simulink model "m02_PMSM_HDL"  (R2023b)
settings: Solver=FixedStepDiscrete  StartTime=0.0  StopTime=0.6  RelTol=1e-3  AbsTol=1e-3
PreLoadFcn:
  | control_data;
  | pmsm_data;
  | 
  | avgFactor = 1;
undefined symbols (not defined in the file): ee_sli_rtmsupport, f1478573793584, f1859323186544, fsw, gcbh, J, Ld, Lq, N, PM, Pmax, Tmax, Ts, Tsc
libraries: hdlssclib x24, simulink x8, SimscapeFPGAHIL_lib x6, fpga_utils_lib x5, hdlsllib x4, eeTransforms x2, eePwmGeneratorTwoLevel x1, eePmsmCurrentController x1, eePmsmCurrentReferenceGen x1, eeVelocityController x1
(part 2 of 3)

== system m02_PMSM_HDL/FPGA Model/HDL Plant/Pejovic HDL Plant/HDL Subsystem/HDL Algorithm/Output ==
  U : Inport
  State : Inport  Port=2
  t : Inport  Port=3
  Mode : Inport  Port=4
  network_outputs : Subsystem
  State Out : Outport  VectorParamsAs1DForOutWhenUnconnected=off
  wires:
  State/1 -> network_outputs/1(x)
  U/1 -> network_outputs/2(u)
  network_outputs/1(vs) -> State Out/1
  t/1 -> network_outputs/3(t)
  Mode/1 -> network_outputs/4(m)

== system m02_PMSM_HDL/FPGA Model/HDL Plant/Pejovic HDL Plant/HDL Subsystem/HDL Algorithm/State Update ==
  U : Inport
  t : Inport  Port=2
  Algebraic Clump1 : Subsystem
  Algebraic Clump2 : Subsystem
  Algebraic Clump3 : Subsystem
  Algebraic Clump4 : Subsystem
  Differential Clump : Subsystem
  Initial Conditions : Subsystem
  State : Outport  VectorParamsAs1DForOutWhenUnconnected=off
  Mode : Outport  Port=2  VectorParamsAs1DForOutWhenUnconnected=off
  wires:
  Initial Conditions/1(State Out) -> Differential Clump/2(State), State/1
  Initial Conditions/2(Mode Out) -> Mode/1, Differential Clump/3(Mode Vector)
  t/1 -> Algebraic Clump1/4(t), Algebraic Clump2/4(t), Algebraic Clump4/4(t), Algebraic Clump3/4(t), Differential Clump/4(t)
  U/1 -> Algebraic Clump1/1(U), Algebraic Clump2/1(U), Algebraic Clump3/1(U), Algebraic Clump4/1(U), Differential Clump/1(U)
  Differential Clump/1(State Out) -> Algebraic Clump1/2(State)
  Differential Clump/2(Mode Vector Out) -> Algebraic Clump1/3(Mode Vector)
  Algebraic Clump1/1(State Out) -> Algebraic Clump2/2(State)
  Algebraic Clump1/2(Mode Vector Out) -> Algebraic Clump2/3(Mode Vector)
  Algebraic Clump2/2(Mode Vector Out) -> Algebraic Clump3/3(Mode Vector)
  Algebraic Clump2/1(State Out) -> Algebraic Clump3/2(State)
  Algebraic Clump3/1(State Out) -> Algebraic Clump4/2(State)
  Algebraic Clump3/2(Mode Vector Out) -> Algebraic Clump4/3(Mode Vector)
  Algebraic Clump4/2(Mode Vector Out) -> Initial Conditions/2(Mode)
  Algebraic Clump4/1(State Out) -> Initial Conditions/1(State)

== system m02_PMSM_HDL/FPGA Model/HDL Plant/Standard HDL Plant/HDL Subsystem/HDL Algorithm/Clock ==
  Delay : Delay  DelayLength=1
  Sample Time : Constant  Value=single(2.5e-06)  OutDataTypeStr=single  SampleTime=2.5e-06
  Sum : Sum  OutDataTypeStr=single
  t : Outport  VectorParamsAs1DForOutWhenUnconnected=off
  wires:
  Sample Time/1 -> Sum/1
  Sum/1 -> Delay/1
  Delay/1 -> t/1, Sum/2

== system m02_PMSM_HDL/FPGA Model/HDL Plant/Standard HDL Plant/HDL Subsystem/HDL Algorithm/Output ==
  U : Inport
  State : Inport  Port=2
  t : Inport  Port=3
  Mode : Inport  Port=4
  network_outputs : Subsystem
  State Out : Outport  VectorParamsAs1DForOutWhenUnconnected=off
  wires:
  Mode/1 -> network_outputs/4(m)
  t/1 -> network_outputs/3(t)
  State/1 -> network_outputs/1(x)
  U/1 -> network_outputs/2(u)
  network_outputs/1(vs) -> State Out/1

== system m02_PMSM_HDL/FPGA Model/HDL Plant/Standard HDL Plant/HDL Subsystem/HDL Algorithm/State Update ==
  U : Inport
  t : Inport  Port=2
  Algebraic Clump1 : Subsystem
  Algebraic Clump2 : Subsystem
  Algebraic Clump3 : Subsystem
  Algebraic Clump4 : Subsystem
  Data Type Conversion : DataTypeConversion  OutDataTypeStr=int32  RndMeth=Nearest  SaturateOnIntegerOverflow=off
  Differential Clump : Subsystem
  Initial Conditions : Subsystem
  Mode Assignment : Assignment  IndexOptions=Index vector (dialog)  Indices="[1  2  4  5  3  6]"  OutputSizes=1
  network_modes : Subsystem
  State : Outport  VectorParamsAs1DForOutWhenUnconnected=off
  Mode : Outport  Port=2  VectorParamsAs1DForOutWhenUnconnected=off
  wires:
  U/1 -> Algebraic Clump3/1(U), Algebraic Clump4/1(U), Algebraic Clump2/1(U), Algebraic Clump1/1(U), network_modes/2(u), Differential Clump/1(U)
  t/1 -> Algebraic Clump3/4(t), Algebraic Clump4/4(t), Algebraic Clump2/4(t), Algebraic Clump1/4(t), network_modes/3(t), Differential Clump/4(t)
  network_modes/1(vs) -> Data Type Conversion/1
  Initial Conditions/1(State Out) -> State/1, Differential Clump/2(State)
  Data Type Conversion/1 -> Mode Assignment/2
  Initial Conditions/2(Mode Out) -> Mode/1, Differential Clump/3(Mode Vector)
  Mode Assignment/1 -> Algebraic Clump1/3(Mode Vector)
  Differential Clump/1(State Out) -> network_modes/1(x), Algebraic Clump1/2(State)
  Differential Clump/2(Mode Vector Out) -> Mode Assignment/1
  Algebraic Clump4/2(Mode Vector Out) -> Initial Conditions/2(Mode)
  Algebraic Clump4/1(State Out) -> Initial Conditions/1(State)
  Algebraic Clump1/1(State Out) -> Algebraic Clump2/2(State)
  Algebraic Clump1/2(Mode Vector Out) -> Algebraic Clump2/3(Mode Vector)
  Algebraic Clump2/2(Mode Vector Out) -> Algebraic Clump3/3(Mode Vector)
  Algebraic Clump2/1(State Out) -> Algebraic Clump3/2(State)
  Algebraic Clump3/1(State Out) -> Algebraic Clump4/2(State)
  Algebraic Clump3/2(Mode Vector Out) -> Algebraic Clump4/3(Mode Vector)

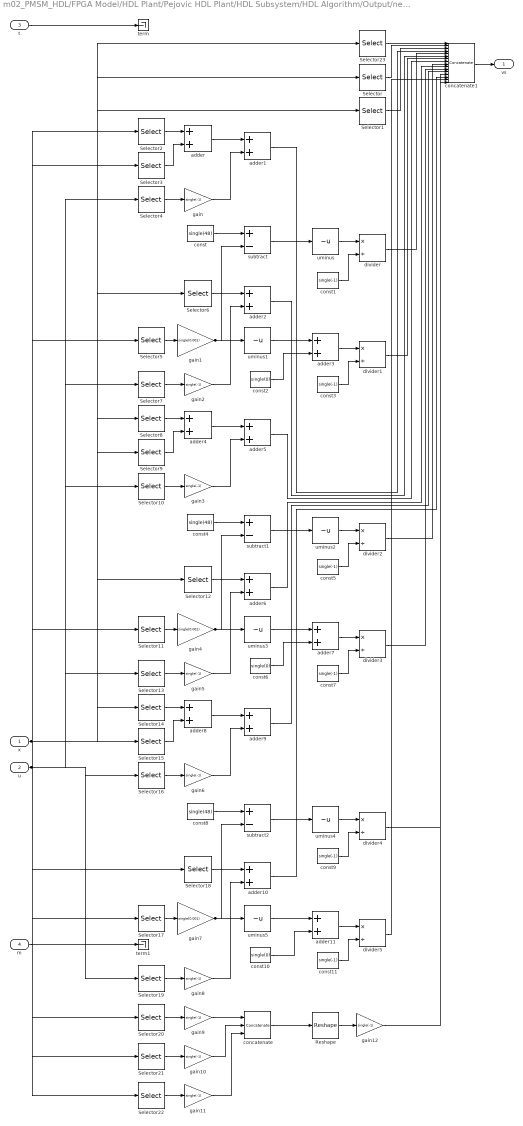
== system m02_PMSM_HDL/FPGA Model/HDL Plant/Pejovic HDL Plant/HDL Subsystem/HDL Algorithm/Output/network_outputs ==
  x : Inport  OutDataTypeStr=single  PortDimensions=[12 1]  SampleTime=2.5e-06
  u : Inport  Port=2  OutDataTypeStr=single  PortDimensions=[6 1]  SampleTime=2.5e-06
  t : Inport  Port=3  OutDataTypeStr=single  SampleTime=2.5e-06
  m : Inport  Port=4  OutDataTypeStr=int32  SampleTime=2.5e-06
  Reshape : Reshape  OutputDimensionality=Row vector (2-D)
  Selector : Selector  SampleTime=2.5e-06  IndexOptions=Index vector (dialog)  Indices=double(7)  OutputSizes=double(0)
  Selector1 : Selector  SampleTime=2.5e-06  IndexOptions=Index vector (dialog)  Indices=double(9)  OutputSizes=double(0)
  Selector{8,10..13} (5 alike) : Selector  SampleTime=2.5e-06  IndexOptions=Index vector (dialog)  Indices=double(2)  OutputSizes=double(0)
  Selector{14,16..19} (5 alike) : Selector  SampleTime=2.5e-06  IndexOptions=Index vector (dialog)  Indices=double(3)  OutputSizes=double(0)
  Selector15 : Selector  SampleTime=2.5e-06  IndexOptions=Index vector (dialog)  Indices=double(6)  OutputSizes=double(0)
  Selector{2,4..7} (5 alike) : Selector  SampleTime=2.5e-06  IndexOptions=Index vector (dialog)  Indices=double(1)  OutputSizes=double(0)
  Selector20 : Selector  SampleTime=2.5e-06  IndexOptions=Index vector (dialog)  Indices=double(4)  OutputSizes=double(0)
  Selector21 : Selector  SampleTime=2.5e-06  IndexOptions=Index vector (dialog)  Indices=double(5)  OutputSizes=double(0)
  Selector22 : Selector  SampleTime=2.5e-06  IndexOptions=Index vector (dialog)  Indices=double(6)  OutputSizes=double(0)
  Selector23 : Selector  SampleTime=2.5e-06  IndexOptions=Index vector (dialog)  Indices=double(8)  OutputSizes=double(0)
  Selector3 : Selector  SampleTime=2.5e-06  IndexOptions=Index vector (dialog)  Indices=double(4)  OutputSizes=double(0)
  Selector9 : Selector  SampleTime=2.5e-06  IndexOptions=Index vector (dialog)  Indices=double(5)  OutputSizes=double(0)
  adder{,1..11} (12 alike) : Sum  OutDataTypeStr=single  AccumDataTypeStr=single  SampleTime=2.5e-06
  concatenate : Concatenate  NumInputs=3  Mode=Multidimensional array
  concatenate1 : Concatenate  NumInputs=16  Mode=Multidimensional array  ConcatenateDimension=2
  const : Constant  Value=single(48)  VectorParams1D=off  OutDataTypeStr=single  SampleTime=2.5e-06
  const{1,3,5,7,9,11} (6 alike) : Constant  Value=single(-1)  VectorParams1D=off  OutDataTypeStr=single  SampleTime=2.5e-06
  const10 : Constant  Value=single(0)  VectorParams1D=off  OutDataTypeStr=single  SampleTime=2.5e-06
  const2 : Constant  Value=single(0)  VectorParams1D=off  OutDataTypeStr=single  SampleTime=2.5e-06
  const4 : Constant  Value=single(48)  VectorParams1D=off  OutDataTypeStr=single  SampleTime=2.5e-06
  const6 : Constant  Value=single(0)  VectorParams1D=off  OutDataTypeStr=single  SampleTime=2.5e-06
  const8 : Constant  Value=single(48)  VectorParams1D=off  OutDataTypeStr=single  SampleTime=2.5e-06
  divider{,1..5} (6 alike) : Product  Inputs=*/  OutDataTypeStr=single  SampleTime=2.5e-06
  gain{,2..3,5..6,8..12} (10 alike) : Gain  Gain=single(-1)  OutDataTypeStr=single  SampleTime=2.5e-06
  gain1 : Gain  Gain=single(0.001)  OutDataTypeStr=single  SampleTime=2.5e-06
  gain4 : Gain  Gain=single(0.001)  OutDataTypeStr=single  SampleTime=2.5e-06
  gain7 : Gain  Gain=single(0.001)  OutDataTypeStr=single  SampleTime=2.5e-06
  subtract : Sum  Inputs=+-  OutDataTypeStr=single  AccumDataTypeStr=single  SampleTime=2.5e-06
  subtract1 : Sum  Inputs=+-  OutDataTypeStr=single  AccumDataTypeStr=single  SampleTime=2.5e-06
  subtract2 : Sum  Inputs=+-  OutDataTypeStr=single  AccumDataTypeStr=single  SampleTime=2.5e-06
  term : Terminator
  term1 : Terminator
  uminus{,1..5} (6 alike) : UnaryMinus  SampleTime=2.5e-06
  vs : Outport  OutDataTypeStr=single  PortDimensions=[1 18]  SampleTime=2.5e-06
  wires:
  Selector20/1 -> gain9/1
  Selector2/1 -> adder/1
  t/1 -> term/1
  u/1 -> Selector19/1, Selector16/1, Selector10/1, Selector7/1, Selector13/1, Selector4/1
  x/1 -> Selector6/1, Selector12/1, Selector1/1, Selector/1, Selector18/1, Selector22/1, Selector21/1, Selector20/1, Selector23/1, Selector15/1, Selector5/1, Selector9/1, Selector14/1, Selector2/1, Selector3/1, Selector11/1, Selector17/1, Selector8/1
  m/1 -> term1/1
  Selector3/1 -> adder/2
  Selector4/1 -> gain/1
  Selector5/1 -> gain1/1
  Selector6/1 -> adder2/1
  Selector7/1 -> gain2/1
  Selector9/1 -> adder4/2
  Selector8/1 -> adder4/1
  Selector11/1 -> gain4/1
  Selector10/1 -> gain3/1
  Selector12/1 -> adder6/1
  Selector13/1 -> gain5/1
  Selector15/1 -> adder8/2
  Selector14/1 -> adder8/1
  Selector17/1 -> gain7/1
  Selector16/1 -> gain6/1
  Selector18/1 -> adder10/1
  Selector19/1 -> gain8/1
  Selector22/1 -> gain11/1
  Selector21/1 -> gain10/1
  adder/1 -> adder1/1
  gain1/1 -> uminus1/1, subtract/2
  gain/1 -> adder1/2
  const1/1 -> divider/2
  const10/1 -> adder11/2
  const/1 -> subtract/1
  gain2/1 -> adder2/2
  adder5/1 -> concatenate1/8
  adder4/1 -> adder5/1
  gain4/1 -> uminus3/1, subtract1/2
  gain3/1 -> adder5/2
  const3/1 -> divider1/2
  const2/1 -> adder3/2
  const4/1 -> subtract1/1
  gain6/1 -> adder9/2
  gain5/1 -> adder6/2
  adder9/1 -> concatenate1/12
  adder8/1 -> adder9/1
  const6/1 -> adder7/2
  const8/1 -> subtract2/1
  gain8/1 -> adder10/2
  gain7/1 -> uminus5/1, subtract2/2
  subtract/1 -> uminus/1
  gain9/1 -> concatenate/1
  gain11/1 -> concatenate/3
  gain10/1 -> concatenate/2
  adder1/1 -> concatenate1/4
  adder2/1 -> concatenate1/6
  uminus2/1 -> divider2/1
  uminus1/1 -> adder3/1
  subtract1/1 -> uminus2/1
  adder6/1 -> concatenate1/10
  uminus3/1 -> adder7/1
  uminus/1 -> divider/1
  subtract2/1 -> uminus4/1
  adder10/1 -> concatenate1/14
  uminus5/1 -> adder11/1
  concatenate/1 -> Reshape/1
  adder3/1 -> divider1/1
  const5/1 -> divider2/2
  adder7/1 -> divider3/1
  const7/1 -> divider3/2
  uminus4/1 -> divider4/1
  const9/1 -> divider4/2
  adder11/1 -> divider5/1
  const11/1 -> divider5/2
  Reshape/1 -> gain12/1
  Selector23/1 -> concatenate1/1
  Selector/1 -> concatenate1/2
  Selector1/1 -> concatenate1/3
  divider/1 -> concatenate1/5
  divider1/1 -> concatenate1/7
  divider2/1 -> concatenate1/9
  divider3/1 -> concatenate1/11
  divider4/1 -> concatenate1/13
  divider5/1 -> concatenate1/15
  gain12/1 -> concatenate1/16
  concatenate1/1 -> vs/1

== system m02_PMSM_HDL/FPGA Model/HDL Plant/Pejovic HDL Plant/HDL Subsystem/HDL Algorithm/State Update/Algebraic Clump1 ==
  U : Inport
  State : Inport  Port=2
  Mode Vector : Inport  Port=3
  t : Inport  Port=4
  Default Index : Constant  Value=fi(0,0,2,0)  SampleTime=2.5e-06
  Multiply F : hdlssclib/NFPSparseConstMultiply  constMatrix=single(f1478573793584.ClumpInfo(1).MdInv)  MatrixType=single  PropDataType=single  defWL=48
  Multiply State : hdlssclib/NFPSparseConstMultiply  constMatrix=single(f1478573793584.ClumpInfo(1).Ad)  MatrixType=single  PropDataType=single  defWL=48
  Out States : Selector  IndexOptions=Index vector (dialog)  Indices="[1  2  3  4]"  OutputSizes=1
  Output Sum : Sum  Inputs=+-
  Owned States : Selector  IndexOptions=Index vector (dialog)  Indices="[1  2  3  4]"  OutputSizes=1
  Ref Inputs : Selector  IndexOptions=Index vector (dialog)  Indices=[1]  OutputSizes=1
  Ref Modes : Selector  IndexOptions=Index vector (dialog)  Indices=[1]  OutputSizes=1
  Ref States : Selector  IndexOptions=Index vector (dialog)  Indices="[7   8   9  10  11  12]"  OutputSizes=1
  State Assign : Assignment  IndexOptions=Index vector (dialog)  Indices="[7   8   9  10]"  OutputSizes=1
  extClump0_F : Subsystem
  transpose : Math  Operator=transpose  SignedPower=on  RndMeth=Zero
  State Out : Outport  VectorParamsAs1DForOutWhenUnconnected=off
  Mode Vector Out : Outport  Port=2  VectorParamsAs1DForOutWhenUnconnected=off
  wires:
  State/1 -> Ref States/1, State Assign/1
  Mode Vector/1 -> Mode Vector Out/1, Ref Modes/1
  U/1 -> Ref Inputs/1
  Ref States/1 -> extClump0_F/1(x), Owned States/1
  Ref Inputs/1 -> extClump0_F/2(u)
  Ref Modes/1 -> extClump0_F/4(m)
  t/1 -> extClump0_F/3(t)
  Owned States/1 -> Multiply State/1
  State Assign/1 -> State Out/1
  Out States/1 -> State Assign/2
  extClump0_F/1(vs) -> transpose/1
  transpose/1 -> Multiply F/1
  Default Index/1 -> Multiply State/2, Multiply F/2
  Multiply State/1 -> Output Sum/1
  Multiply F/1 -> Output Sum/2
  Output Sum/1 -> Out States/1

== system m02_PMSM_HDL/FPGA Model/HDL Plant/Pejovic HDL Plant/HDL Subsystem/HDL Algorithm/State Update/Algebraic Clump2 ==
  U : Inport
  State : Inport  Port=2
  Mode Vector : Inport  Port=3
  t : Inport  Port=4
  Default Index : Constant  Value=fi(0,0,2,0)  SampleTime=2.5e-06
  Multiply F : hdlssclib/NFPSparseConstMultiply  constMatrix=single(f1478573793584.ClumpInfo(2).MdInv)  MatrixType=single  PropDataType=single  defWL=48
  Multiply State : hdlssclib/NFPSparseConstMultiply  constMatrix=single(f1478573793584.ClumpInfo(2).Ad)  MatrixType=single  PropDataType=single  defWL=48
  Out States : Selector  IndexOptions=Index vector (dialog)  Indices="[1  2]"  OutputSizes=1
  Output Sum : Sum  Inputs=+-
  Owned States : Selector  IndexOptions=Index vector (dialog)  Indices="[1  2]"  OutputSizes=1
  Ref Inputs : Selector  IndexOptions=Index vector (dialog)  Indices="[6  3]"  OutputSizes=1
  Ref Modes : Selector  IndexOptions=Index vector (dialog)  Indices=[1]  OutputSizes=1
  Ref States : Selector  IndexOptions=Index vector (dialog)  Indices="[3   6  10  11  12]"  OutputSizes=1
  State Assign : Assignment  IndexOptions=Index vector (dialog)  Indices="[3  6]"  OutputSizes=1
  extClump1_F : Subsystem
  transpose : Math  Operator=transpose  SignedPower=on  RndMeth=Zero
  State Out : Outport  VectorParamsAs1DForOutWhenUnconnected=off
  Mode Vector Out : Outport  Port=2  VectorParamsAs1DForOutWhenUnconnected=off
  wires:
  State/1 -> Ref States/1, State Assign/1
  Out States/1 -> State Assign/2
  U/1 -> Ref Inputs/1
  Mode Vector/1 -> Mode Vector Out/1, Ref Modes/1
  Ref States/1 -> extClump1_F/1(x), Owned States/1
  Ref Inputs/1 -> extClump1_F/2(u)
  Ref Modes/1 -> extClump1_F/4(m)
  t/1 -> extClump1_F/3(t)
  Owned States/1 -> Multiply State/1
  extClump1_F/1(vs) -> transpose/1
  transpose/1 -> Multiply F/1
  Default Index/1 -> Multiply State/2, Multiply F/2
  Multiply State/1 -> Output Sum/1
  Multiply F/1 -> Output Sum/2
  Output Sum/1 -> Out States/1
  State Assign/1 -> State Out/1

== system m02_PMSM_HDL/FPGA Model/HDL Plant/Pejovic HDL Plant/HDL Subsystem/HDL Algorithm/State Update/Algebraic Clump3 ==
  U : Inport
  State : Inport  Port=2
  Mode Vector : Inport  Port=3
  t : Inport  Port=4
  Default Index : Constant  Value=fi(0,0,2,0)  SampleTime=2.5e-06
  Multiply F : hdlssclib/NFPSparseConstMultiply  constMatrix=single(f1478573793584.ClumpInfo(3).MdInv)  MatrixType=single  PropDataType=single  defWL=48
  Multiply State : hdlssclib/NFPSparseConstMultiply  constMatrix=single(f1478573793584.ClumpInfo(3).Ad)  MatrixType=single  PropDataType=single  defWL=48
  Out States : Selector  IndexOptions=Index vector (dialog)  Indices="[1  2]"  OutputSizes=1
  Output Sum : Sum  Inputs=+-
  Owned States : Selector  IndexOptions=Index vector (dialog)  Indices="[1  2]"  OutputSizes=1
  Ref Inputs : Selector  IndexOptions=Index vector (dialog)  Indices="[5  2]"  OutputSizes=1
  Ref Modes : Selector  IndexOptions=Index vector (dialog)  Indices=[1]  OutputSizes=1
  Ref States : Selector  IndexOptions=Index vector (dialog)  Indices="[2   5  10  11  12]"  OutputSizes=1
  State Assign : Assignment  IndexOptions=Index vector (dialog)  Indices="[2  5]"  OutputSizes=1
  extClump2_F : Subsystem
  transpose : Math  Operator=transpose  SignedPower=on  RndMeth=Zero
  State Out : Outport  VectorParamsAs1DForOutWhenUnconnected=off
  Mode Vector Out : Outport  Port=2  VectorParamsAs1DForOutWhenUnconnected=off
  wires:
  Output Sum/1 -> Out States/1
  Default Index/1 -> Multiply State/2, Multiply F/2
  State/1 -> State Assign/1, Ref States/1
  State Assign/1 -> State Out/1
  U/1 -> Ref Inputs/1
  Ref Inputs/1 -> extClump2_F/2(u)
  Mode Vector/1 -> Ref Modes/1, Mode Vector Out/1
  Ref States/1 -> extClump2_F/1(x), Owned States/1
  Owned States/1 -> Multiply State/1
  Ref Modes/1 -> extClump2_F/4(m)
  t/1 -> extClump2_F/3(t)
  extClump2_F/1(vs) -> transpose/1
  transpose/1 -> Multiply F/1
  Multiply State/1 -> Output Sum/1
  Multiply F/1 -> Output Sum/2
  Out States/1 -> State Assign/2

== system m02_PMSM_HDL/FPGA Model/HDL Plant/Pejovic HDL Plant/HDL Subsystem/HDL Algorithm/State Update/Algebraic Clump4 ==
  U : Inport
  State : Inport  Port=2
  Mode Vector : Inport  Port=3
  t : Inport  Port=4
  Default Index : Constant  Value=fi(0,0,2,0)  SampleTime=2.5e-06
  Multiply F : hdlssclib/NFPSparseConstMultiply  constMatrix=single(f1478573793584.ClumpInfo(4).MdInv)  MatrixType=single  PropDataType=single  defWL=48
  Multiply State : hdlssclib/NFPSparseConstMultiply  constMatrix=single(f1478573793584.ClumpInfo(4).Ad)  MatrixType=single  PropDataType=single  defWL=48
  Out States : Selector  IndexOptions=Index vector (dialog)  Indices="[1  2]"  OutputSizes=1
  Output Sum : Sum  Inputs=+-
  Owned States : Selector  IndexOptions=Index vector (dialog)  Indices="[1  2]"  OutputSizes=1
  Ref Inputs : Selector  IndexOptions=Index vector (dialog)  Indices="[4  1]"  OutputSizes=1
  Ref Modes : Selector  IndexOptions=Index vector (dialog)  Indices=[1]  OutputSizes=1
  Ref States : Selector  IndexOptions=Index vector (dialog)  Indices="[1   4  10  11  12]"  OutputSizes=1
  State Assign : Assignment  IndexOptions=Index vector (dialog)  Indices="[1  4]"  OutputSizes=1
  extClump3_F : Subsystem
  transpose : Math  Operator=transpose  SignedPower=on  RndMeth=Zero
  State Out : Outport  VectorParamsAs1DForOutWhenUnconnected=off
  Mode Vector Out : Outport  Port=2  VectorParamsAs1DForOutWhenUnconnected=off
  wires:
  Ref States/1 -> Owned States/1, extClump3_F/1(x)
  State/1 -> State Assign/1, Ref States/1
  Mode Vector/1 -> Mode Vector Out/1, Ref Modes/1
  U/1 -> Ref Inputs/1
  Ref Inputs/1 -> extClump3_F/2(u)
  Ref Modes/1 -> extClump3_F/4(m)
  t/1 -> extClump3_F/3(t)
  Owned States/1 -> Multiply State/1
  extClump3_F/1(vs) -> transpose/1
  transpose/1 -> Multiply F/1
  Default Index/1 -> Multiply State/2, Multiply F/2
  Multiply State/1 -> Output Sum/1
  Multiply F/1 -> Output Sum/2
  Output Sum/1 -> Out States/1
  Out States/1 -> State Assign/2
  State Assign/1 -> State Out/1

== system m02_PMSM_HDL/FPGA Model/HDL Plant/Pejovic HDL Plant/HDL Subsystem/HDL Algorithm/State Update/Differential Clump ==
  U : Inport
  State : Inport  Port=2
  Mode Vector : Inport  Port=3
  t : Inport  Port=4
  Default Index : Constant  Value=fi(0,0,2,0)  SampleTime=2.5e-06
  Input Delay : Delay  DelayLength=1
  Multiply F : hdlssclib/NFPSparseConstMultiply  constMatrix=single(f1478573793584.DiffClumpInfo.MdInv)  MatrixType=single  PropDataType=single  defWL=48
  Output Sum : Sum  Inputs=+-
  Owned States : Selector  IndexOptions=Index vector (dialog)  Indices="[11  12]"  OutputSizes=1
  State Assign : Assignment  IndexOptions=Index vector (dialog)  Indices="[11  12]"  OutputSizes=1
  diffClump_F : Subsystem
  t Delay : Delay  DelayLength=1
  transpose : Math  Operator=transpose  SignedPower=on  RndMeth=Zero
  State Out : Outport  VectorParamsAs1DForOutWhenUnconnected=off
  Mode Vector Out : Outport  Port=2  VectorParamsAs1DForOutWhenUnconnected=off
  wires:
  Mode Vector/1 -> Mode Vector Out/1, diffClump_F/4(m)
  U/1 -> Input Delay/1
  State/1 -> Owned States/1, State Assign/1, diffClump_F/1(x)
  t/1 -> t Delay/1
  Input Delay/1 -> diffClump_F/2(u)
  t Delay/1 -> diffClump_F/3(t)
  diffClump_F/1(vs) -> transpose/1
  transpose/1 -> Multiply F/1
  Output Sum/1 -> State Assign/2
  Default Index/1 -> Multiply F/2
  Owned States/1 -> Output Sum/1
  Multiply F/1 -> Output Sum/2
  State Assign/1 -> State Out/1

== system m02_PMSM_HDL/FPGA Model/HDL Plant/Pejovic HDL Plant/HDL Subsystem/HDL Algorithm/State Update/Initial Conditions ==
  State : Inport
  Mode : Inport  Port=2
  Constant : Constant  Value=single(f1478573793584.IC.X)  SampleTime=2.5e-06
  Constant1 : Constant  Value=f1478573793584.IM  SampleTime=2.5e-06
  Delay{,1..3} (4 alike) : Delay  DelayLength=1
  Switch : Switch  Criteria=u2 ~= 0  OutDataTypeStr=single  SaturateOnIntegerOverflow=off  InputSameDT=off
  Switch1 : Switch  Criteria=u2 ~= 0  OutDataTypeStr=int32  SaturateOnIntegerOverflow=off  InputSameDT=off
  Valid Out : Constant  OutDataTypeStr=boolean  SampleTime=2.5e-06
  State Out : Outport  VectorParamsAs1DForOutWhenUnconnected=off
  Mode Out : Outport  Port=2  VectorParamsAs1DForOutWhenUnconnected=off
  wires:
  Valid Out/1 -> Delay2/1
  Delay2/1 -> Delay3/1, Switch1/2
  Delay3/1 -> Switch/2
  State/1 -> Delay/1
  Delay/1 -> Switch/1
  Constant/1 -> Switch/3
  Switch/1 -> State Out/1
  Mode/1 -> Delay1/1
  Delay1/1 -> Switch1/1
  Constant1/1 -> Switch1/3
  Switch1/1 -> Mode Out/1

== system m02_PMSM_HDL/FPGA Model/HDL Plant/Standard HDL Plant/HDL Subsystem/HDL Algorithm/Output/network_outputs ==
  x : Inport  OutDataTypeStr=single  PortDimensions=[15 1]  SampleTime=2.5e-06
  u : Inport  Port=2  OutDataTypeStr=single  PortDimensions=[6 1]  SampleTime=2.5e-06
  t : Inport  Port=3  OutDataTypeStr=single  SampleTime=2.5e-06
  m : Inport  Port=4  OutDataTypeStr=int32  PortDimensions=[6 1]  SampleTime=2.5e-06
  Reshape : Reshape  OutputDimensionality=Row vector (2-D)
  Selector : Selector  IndexOptions=Index vector (dialog)  Indices=double(7)  OutputSizes=double(0)
  Selector1 : Selector  IndexOptions=Index vector (dialog)  Indices=double(9)  OutputSizes=double(0)
  Selector2 : Selector  IndexOptions=Index vector (dialog)  Indices=double(4)  OutputSizes=double(0)
  Selector3 : Selector  IndexOptions=Index vector (dialog)  Indices=double(5)  OutputSizes=double(0)
  Selector4 : Selector  IndexOptions=Index vector (dialog)  Indices=double(6)  OutputSizes=double(0)
  Selector5 : Selector  IndexOptions=Index vector (dialog)  Indices=double(8)  OutputSizes=double(0)
  concatenate : Concatenate  NumInputs=3  Mode=Multidimensional array
  concatenate1 : Concatenate  NumInputs=4  Mode=Multidimensional array  ConcatenateDimension=2
  gain{,1..3} (4 alike) : Gain  Gain=single(-1)  OutDataTypeStr=single  SampleTime=2.5e-06
  term : Terminator
  term1 : Terminator
  term2 : Terminator
  vs : Outport  OutDataTypeStr=single  PortDimensions=[1 6]  SampleTime=2.5e-06
  wires:
  Reshape/1 -> gain3/1
  m/1 -> term2/1
  t/1 -> term1/1
  x/1 -> Selector/1, Selector3/1, Selector2/1, Selector5/1, Selector4/1, Selector1/1
  u/1 -> term/1
  Selector2/1 -> gain/1
  Selector3/1 -> gain1/1
  Selector5/1 -> concatenate1/1
  Selector4/1 -> gain2/1
  concatenate1/1 -> vs/1
  gain/1 -> concatenate/1
  gain2/1 -> concatenate/3
  gain1/1 -> concatenate/2
  Selector1/1 -> concatenate1/3
  Selector/1 -> concatenate1/2
  concatenate/1 -> Reshape/1
  gain3/1 -> concatenate1/4

== system m02_PMSM_HDL/FPGA Model/HDL Plant/Standard HDL Plant/HDL Subsystem/HDL Algorithm/State Update/Algebraic Clump1 ==
  U : Inport
  State : Inport  Port=2
  Mode Vector : Inport  Port=3
  t : Inport  Port=4
  Default Index : Constant  Value=fi(0,0,2,0)  SampleTime=2.5e-06
  Multiply F : hdlssclib/NFPSparseConstMultiply  constMatrix=single(f1859323186544.ClumpInfo(1).MdInv)  MatrixType=single  PropDataType=single  defWL=48
  Multiply State : hdlssclib/NFPSparseConstMultiply  constMatrix=single(f1859323186544.ClumpInfo(1).Ad)  MatrixType=single  PropDataType=single  defWL=48
  Out States : Selector  IndexOptions=Index vector (dialog)  Indices="[1  2  3  4]"  OutputSizes=1
  Output Sum : Sum  Inputs=+-
  Owned States : Selector  IndexOptions=Index vector (dialog)  Indices="[1  2  3  4]"  OutputSizes=1
  Ref Inputs : Selector  IndexOptions=Index vector (dialog)  Indices=[1]  OutputSizes=1
  Ref Modes : Selector  IndexOptions=Index vector (dialog)  Indices=[1]  OutputSizes=1
  Ref States : Selector  IndexOptions=Index vector (dialog)  Indices="[7   8   9  13  14  15]"  OutputSizes=1
  State Assign : Assignment  IndexOptions=Index vector (dialog)  Indices="[7   8   9  13]"  OutputSizes=1
  extClump0_F : Subsystem
  transpose : Math  Operator=transpose  SignedPower=on  RndMeth=Zero
  State Out : Outport  VectorParamsAs1DForOutWhenUnconnected=off
  Mode Vector Out : Outport  Port=2  VectorParamsAs1DForOutWhenUnconnected=off
  wires:
  State/1 -> State Assign/1, Ref States/1
  Ref Modes/1 -> extClump0_F/4(m)
  U/1 -> Ref Inputs/1
  Ref Inputs/1 -> extClump0_F/2(u)
  transpose/1 -> Multiply F/1
  Mode Vector/1 -> Mode Vector Out/1, Ref Modes/1
  Ref States/1 -> extClump0_F/1(x), Owned States/1
  t/1 -> extClump0_F/3(t)
  Owned States/1 -> Multiply State/1
  extClump0_F/1(vs) -> transpose/1
  Default Index/1 -> Multiply State/2, Multiply F/2
  Multiply State/1 -> Output Sum/1
  Multiply F/1 -> Output Sum/2
  Output Sum/1 -> Out States/1
  Out States/1 -> State Assign/2
  State Assign/1 -> State Out/1

== system m02_PMSM_HDL/FPGA Model/HDL Plant/Standard HDL Plant/HDL Subsystem/HDL Algorithm/State Update/Algebraic Clump2 ==
  U : Inport
  State : Inport  Port=2
  Mode Vector : Inport  Port=3
  t : Inport  Port=4
  Mode Vector To Index : Subsystem
  Mode Vector Type Conversion : Subsystem
  Multiply F : hdlssclib/NFPSparseConstMultiply  constMatrix=single(f1859323186544.ClumpInfo(2).MdInv)  MatrixType=single  PropDataType=single  defWL=48
  Multiply State : hdlssclib/NFPSparseConstMultiply  constMatrix=single(f1859323186544.ClumpInfo(2).Ad)  MatrixType=single  PropDataType=single  defWL=48
  Out States : Selector  IndexOptions=Index vector (dialog)  Indices="[1  2  3]"  OutputSizes=1
  Output Sum : Sum  Inputs=+-
  Owned States : Selector  IndexOptions=Index vector (dialog)  Indices="[1  2  3]"  OutputSizes=1
  Ref Inputs : Selector  IndexOptions=Index vector (dialog)  Indices="[5  6]"  OutputSizes=1
  Ref Modes : Selector  IndexOptions=Index vector (dialog)  Indices="[5  6]"  OutputSizes=1
  Ref States : Selector  IndexOptions=Index vector (dialog)  Indices="[12   3   6  13  14  15]"  OutputSizes=1
  Selector : Selector  IndexOptions=Index vector (dialog)  Indices="[5  6]"  OutputSizes=1
  State Assign : Assignment  IndexOptions=Index vector (dialog)  Indices="[12   3   6]"  OutputSizes=1
  extClump1_F : Subsystem
  transpose : Math  Operator=transpose  SignedPower=on  RndMeth=Zero
  State Out : Outport  VectorParamsAs1DForOutWhenUnconnected=off
  Mode Vector Out : Outport  Port=2  VectorParamsAs1DForOutWhenUnconnected=off
  wires:
  State/1 -> State Assign/1, Ref States/1
  Mode Vector/1 -> Selector/1, Mode Vector Out/1, Ref Modes/1
  U/1 -> Ref Inputs/1
  Ref States/1 -> Owned States/1, extClump1_F/1(x)
  Ref Modes/1 -> extClump1_F/4(m)
  Owned States/1 -> Multiply State/1
  Ref Inputs/1 -> extClump1_F/2(u)
  t/1 -> extClump1_F/3(t)
  State Assign/1 -> State Out/1
  Selector/1 -> Mode Vector Type Conversion/1(Mode vec)
  extClump1_F/1(vs) -> transpose/1
  Mode Vector To Index/1(Out1) -> Multiply State/2, Multiply F/2
  Mode Vector Type Conversion/1(Out1) -> Mode Vector To Index/1(In1)
  transpose/1 -> Multiply F/1
  Out States/1 -> State Assign/2
  Multiply State/1 -> Output Sum/1
  Multiply F/1 -> Output Sum/2
  Output Sum/1 -> Out States/1

== system m02_PMSM_HDL/FPGA Model/HDL Plant/Standard HDL Plant/HDL Subsystem/HDL Algorithm/State Update/Algebraic Clump3 ==
  U : Inport
  State : Inport  Port=2
  Mode Vector : Inport  Port=3
  t : Inport  Port=4
  Mode Vector To Index : Subsystem
  Mode Vector Type Conversion : Subsystem
  Multiply F : hdlssclib/NFPSparseConstMultiply  constMatrix=single(f1859323186544.ClumpInfo(3).MdInv)  MatrixType=single  PropDataType=single  defWL=48
  Multiply State : hdlssclib/NFPSparseConstMultiply  constMatrix=single(f1859323186544.ClumpInfo(3).Ad)  MatrixType=single  PropDataType=single  defWL=48
  Out States : Selector  IndexOptions=Index vector (dialog)  Indices="[1  2  3]"  OutputSizes=1
  Output Sum : Sum  Inputs=+-
  Owned States : Selector  IndexOptions=Index vector (dialog)  Indices="[1  2  3]"  OutputSizes=1
  Ref Inputs : Selector  IndexOptions=Index vector (dialog)  Indices="[3  4]"  OutputSizes=1
  Ref Modes : Selector  IndexOptions=Index vector (dialog)  Indices="[3  4]"  OutputSizes=1
  Ref States : Selector  IndexOptions=Index vector (dialog)  Indices="[11   2   5  13  14  15]"  OutputSizes=1
  Selector : Selector  IndexOptions=Index vector (dialog)  Indices="[3  4]"  OutputSizes=1
  State Assign : Assignment  IndexOptions=Index vector (dialog)  Indices="[11   2   5]"  OutputSizes=1
  extClump2_F : Subsystem
  transpose : Math  Operator=transpose  SignedPower=on  RndMeth=Zero
  State Out : Outport  VectorParamsAs1DForOutWhenUnconnected=off
  Mode Vector Out : Outport  Port=2  VectorParamsAs1DForOutWhenUnconnected=off
  wires:
  State/1 -> State Assign/1, Ref States/1
  U/1 -> Ref Inputs/1
  Ref States/1 -> Owned States/1, extClump2_F/1(x)
  Selector/1 -> Mode Vector Type Conversion/1(Mode vec)
  Mode Vector/1 -> Selector/1, Mode Vector Out/1, Ref Modes/1
  t/1 -> extClump2_F/3(t)
  Ref Inputs/1 -> extClump2_F/2(u)
  Ref Modes/1 -> extClump2_F/4(m)
  extClump2_F/1(vs) -> transpose/1
  Mode Vector Type Conversion/1(Out1) -> Mode Vector To Index/1(In1)
  Output Sum/1 -> Out States/1
  Owned States/1 -> Multiply State/1
  State Assign/1 -> State Out/1
  transpose/1 -> Multiply F/1
  Mode Vector To Index/1(Out1) -> Multiply State/2, Multiply F/2
  Multiply F/1 -> Output Sum/2
  Multiply State/1 -> Output Sum/1
  Out States/1 -> State Assign/2

== system m02_PMSM_HDL/FPGA Model/HDL Plant/Standard HDL Plant/HDL Subsystem/HDL Algorithm/State Update/Algebraic Clump4 ==
  U : Inport
  State : Inport  Port=2
  Mode Vector : Inport  Port=3
  t : Inport  Port=4
  Mode Vector To Index : Subsystem
  Mode Vector Type Conversion : Subsystem
  Multiply F : hdlssclib/NFPSparseConstMultiply  constMatrix=single(f1859323186544.ClumpInfo(4).MdInv)  MatrixType=single  PropDataType=single  defWL=48
  Multiply State : hdlssclib/NFPSparseConstMultiply  constMatrix=single(f1859323186544.ClumpInfo(4).Ad)  MatrixType=single  PropDataType=single  defWL=48
  Out States : Selector  IndexOptions=Index vector (dialog)  Indices="[1  2  3]"  OutputSizes=1
  Output Sum : Sum  Inputs=+-
  Owned States : Selector  IndexOptions=Index vector (dialog)  Indices="[1  2  3]"  OutputSizes=1
  Ref Inputs : Selector  IndexOptions=Index vector (dialog)  Indices="[1  2]"  OutputSizes=1
  Ref Modes : Selector  IndexOptions=Index vector (dialog)  Indices="[1  2]"  OutputSizes=1
  Ref States : Selector  IndexOptions=Index vector (dialog)  Indices="[10   1   4  13  14  15]"  OutputSizes=1
  Selector : Selector  IndexOptions=Index vector (dialog)  Indices="[1  2]"  OutputSizes=1
  State Assign : Assignment  IndexOptions=Index vector (dialog)  Indices="[10   1   4]"  OutputSizes=1
  extClump3_F : Subsystem
  transpose : Math  Operator=transpose  SignedPower=on  RndMeth=Zero
  State Out : Outport  VectorParamsAs1DForOutWhenUnconnected=off
  Mode Vector Out : Outport  Port=2  VectorParamsAs1DForOutWhenUnconnected=off
  wires:
  Owned States/1 -> Multiply State/1
  Ref Inputs/1 -> extClump3_F/2(u)
  State/1 -> Ref States/1, State Assign/1
  Mode Vector/1 -> Mode Vector Out/1, Ref Modes/1, Selector/1
  U/1 -> Ref Inputs/1
  Ref States/1 -> Owned States/1, extClump3_F/1(x)
  Ref Modes/1 -> extClump3_F/4(m)
  t/1 -> extClump3_F/3(t)
  State Assign/1 -> State Out/1
  Selector/1 -> Mode Vector Type Conversion/1(Mode vec)
  extClump3_F/1(vs) -> transpose/1
  Mode Vector To Index/1(Out1) -> Multiply State/2, Multiply F/2
  Mode Vector Type Conversion/1(Out1) -> Mode Vector To Index/1(In1)
  transpose/1 -> Multiply F/1
  Out States/1 -> State Assign/2
  Multiply State/1 -> Output Sum/1
  Multiply F/1 -> Output Sum/2
  Output Sum/1 -> Out States/1

== system m02_PMSM_HDL/FPGA Model/HDL Plant/Standard HDL Plant/HDL Subsystem/HDL Algorithm/State Update/Differential Clump ==
  U : Inport
  State : Inport  Port=2
  Mode Vector : Inport  Port=3
  t : Inport  Port=4
  Default Index : Constant  Value=fi(0,0,2,0)  SampleTime=2.5e-06
  Input Delay : Delay  DelayLength=1
  Multiply F : hdlssclib/NFPSparseConstMultiply  constMatrix=single(f1859323186544.DiffClumpInfo.MdInv)  MatrixType=single  PropDataType=single  defWL=48
  Output Sum : Sum  Inputs=+-
  Owned States : Selector  IndexOptions=Index vector (dialog)  Indices="[14  15]"  OutputSizes=1
  State Assign : Assignment  IndexOptions=Index vector (dialog)  Indices="[14  15]"  OutputSizes=1
  diffClump_F : Subsystem
  t Delay : Delay  DelayLength=1
  transpose : Math  Operator=transpose  SignedPower=on  RndMeth=Zero
  State Out : Outport  VectorParamsAs1DForOutWhenUnconnected=off
  Mode Vector Out : Outport  Port=2  VectorParamsAs1DForOutWhenUnconnected=off
  wires:
  U/1 -> Input Delay/1
  t Delay/1 -> diffClump_F/3(t)
  t/1 -> t Delay/1
  State/1 -> Owned States/1, State Assign/1, diffClump_F/1(x)
  Mode Vector/1 -> Mode Vector Out/1, diffClump_F/4(m)
  Input Delay/1 -> diffClump_F/2(u)
  diffClump_F/1(vs) -> transpose/1
  transpose/1 -> Multiply F/1
  Default Index/1 -> Multiply F/2
  Owned States/1 -> Output Sum/1
  Multiply F/1 -> Output Sum/2
  Output Sum/1 -> State Assign/2
  State Assign/1 -> State Out/1

== system m02_PMSM_HDL/FPGA Model/HDL Plant/Standard HDL Plant/HDL Subsystem/HDL Algorithm/State Update/Initial Conditions ==
  State : Inport
  Mode : Inport  Port=2
  Constant : Constant  Value=single(f1859323186544.IC.X)  SampleTime=2.5e-06
  Constant1 : Constant  Value=f1859323186544.IM  SampleTime=2.5e-06
  Delay{,1..3} (4 alike) : Delay  DelayLength=1
  Switch : Switch  Criteria=u2 ~= 0  OutDataTypeStr=single  SaturateOnIntegerOverflow=off  InputSameDT=off
  Switch1 : Switch  Criteria=u2 ~= 0  OutDataTypeStr=int32  SaturateOnIntegerOverflow=off  InputSameDT=off
  Valid Out : Constant  OutDataTypeStr=boolean  SampleTime=2.5e-06
  State Out : Outport  VectorParamsAs1DForOutWhenUnconnected=off
  Mode Out : Outport  Port=2  VectorParamsAs1DForOutWhenUnconnected=off
  wires:
  Valid Out/1 -> Delay2/1
  Delay2/1 -> Delay3/1, Switch1/2
  Delay3/1 -> Switch/2
  State/1 -> Delay/1
  Delay/1 -> Switch/1
  Constant/1 -> Switch/3
  Switch/1 -> State Out/1
  Mode/1 -> Delay1/1
  Delay1/1 -> Switch1/1
  Constant1/1 -> Switch1/3
  Switch1/1 -> Mode Out/1

== system m02_PMSM_HDL/FPGA Model/HDL Plant/Standard HDL Plant/HDL Subsystem/HDL Algorithm/State Update/network_modes ==
  x : Inport  OutDataTypeStr=single  PortDimensions=[15 1]  SampleTime=2.5e-06
  u : Inport  Port=2  OutDataTypeStr=single  PortDimensions=[6 1]  SampleTime=2.5e-06
  t : Inport  Port=3  OutDataTypeStr=single  SampleTime=2.5e-06
  Selector : Selector  IndexOptions=Index vector (dialog)  Indices=double(1)  OutputSizes=double(0)
  Selector1 : Selector  IndexOptions=Index vector (dialog)  Indices=double(2)  OutputSizes=double(0)
  Selector2 : Selector  IndexOptions=Index vector (dialog)  Indices=double(4)  OutputSizes=double(0)
  Selector3 : Selector  IndexOptions=Index vector (dialog)  Indices=double(5)  OutputSizes=double(0)
  Selector4 : Selector  IndexOptions=Index vector (dialog)  Indices=double(3)  OutputSizes=double(0)
  Selector5 : Selector  IndexOptions=Index vector (dialog)  Indices=double(6)  OutputSizes=double(0)
  compare{,1..5} (6 alike) : simulink/Logic and Bit Operations/Compare To Constant  relop=>  const=single(0.5)  OutDataTypeStr=boolean
  concatenate : Concatenate  NumInputs=6  ConcatenateDimension=2
  term : Terminator
  term1 : Terminator
  vs : Outport  OutDataTypeStr=boolean  PortDimensions=[1 6]  SampleTime=2.5e-06
  wires:
  x/1 -> term/1
  t/1 -> term1/1
  Selector/1 -> compare/1
  compare4/1 -> concatenate/5
  Selector4/1 -> compare4/1
  u/1 -> Selector4/1, Selector/1, Selector2/1, Selector1/1, Selector3/1, Selector5/1
  Selector3/1 -> compare3/1
  Selector1/1 -> compare1/1
  Selector2/1 -> compare2/1
  compare5/1 -> concatenate/6
  Selector5/1 -> compare5/1
  compare/1 -> concatenate/1
  compare1/1 -> concatenate/2
  compare2/1 -> concatenate/3
  compare3/1 -> concatenate/4
  concatenate/1 -> vs/1

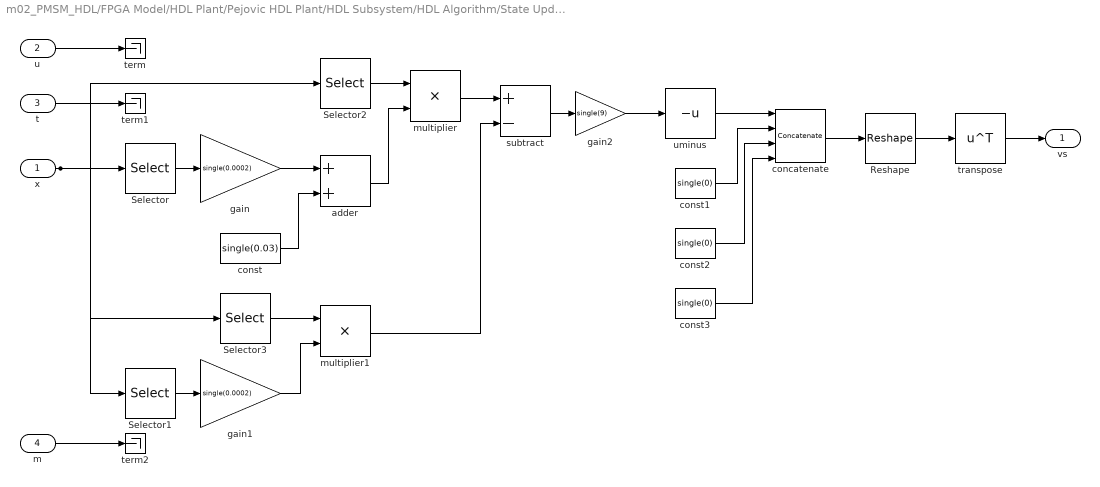
== system m02_PMSM_HDL/FPGA Model/HDL Plant/Pejovic HDL Plant/HDL Subsystem/HDL Algorithm/State Update/Algebraic Clump1/extClump0_F ==
  x : Inport  OutDataTypeStr=single  PortDimensions=[6 1]  SampleTime=2.5e-06
  u : Inport  Port=2  OutDataTypeStr=single  SampleTime=2.5e-06
  t : Inport  Port=3  OutDataTypeStr=single  SampleTime=2.5e-06
  m : Inport  Port=4  OutDataTypeStr=int32  SampleTime=2.5e-06
  Reshape : Reshape  OutputDimensionality=Column vector (2-D)
  Selector : Selector  SampleTime=2.5e-06  IndexOptions=Index vector (dialog)  Indices=double(5)  OutputSizes=double(0)
  Selector1 : Selector  SampleTime=2.5e-06  IndexOptions=Index vector (dialog)  Indices=double(6)  OutputSizes=double(0)
  Selector2 : Selector  SampleTime=2.5e-06  IndexOptions=Index vector (dialog)  Indices=double(6)  OutputSizes=double(0)
  Selector3 : Selector  SampleTime=2.5e-06  IndexOptions=Index vector (dialog)  Indices=double(5)  OutputSizes=double(0)
  adder : Sum  OutDataTypeStr=single  AccumDataTypeStr=single  SampleTime=2.5e-06
  concatenate : Concatenate  NumInputs=4  Mode=Multidimensional array
  const : Constant  Value=single(0.03)  VectorParams1D=off  OutDataTypeStr=single  SampleTime=2.5e-06
  const1 : Constant  Value=single(0)  VectorParams1D=off  OutDataTypeStr=single  SampleTime=2.5e-06
  const2 : Constant  Value=single(0)  VectorParams1D=off  OutDataTypeStr=single  SampleTime=2.5e-06
  const3 : Constant  Value=single(0)  VectorParams1D=off  OutDataTypeStr=single  SampleTime=2.5e-06
  gain : Gain  Gain=single(0.0002)  OutDataTypeStr=single  SampleTime=2.5e-06
  gain1 : Gain  Gain=single(0.0002)  OutDataTypeStr=single  SampleTime=2.5e-06
  gain2 : Gain  Gain=single(9)  OutDataTypeStr=single  SampleTime=2.5e-06
  multiplier : Product  Inputs=**  OutDataTypeStr=single  SampleTime=2.5e-06
  multiplier1 : Product  Inputs=**  OutDataTypeStr=single  SampleTime=2.5e-06
  subtract : Sum  Inputs=+-  OutDataTypeStr=single  AccumDataTypeStr=single  SampleTime=2.5e-06
  term : Terminator
  term1 : Terminator
  term2 : Terminator
  transpose : Math  Operator=transpose
  uminus : UnaryMinus  SampleTime=2.5e-06
  vs : Outport  OutDataTypeStr=single  PortDimensions=[1 4]  SampleTime=2.5e-06
  wires:
  u/1 -> term/1
  x/1 -> Selector2/1, Selector/1, Selector1/1, Selector3/1
  t/1 -> term1/1
  m/1 -> term2/1
  Reshape/1 -> transpose/1
  Selector/1 -> gain/1
  Selector2/1 -> multiplier/1
  Selector1/1 -> gain1/1
  const3/1 -> concatenate/4
  const2/1 -> concatenate/3
  gain/1 -> adder/1
  concatenate/1 -> Reshape/1
  const1/1 -> concatenate/2
  const/1 -> adder/2
  Selector3/1 -> multiplier1/1
  gain2/1 -> uminus/1
  gain1/1 -> multiplier1/2
  adder/1 -> multiplier/2
  multiplier1/1 -> subtract/2
  multiplier/1 -> subtract/1
  transpose/1 -> vs/1
  subtract/1 -> gain2/1
  uminus/1 -> concatenate/1

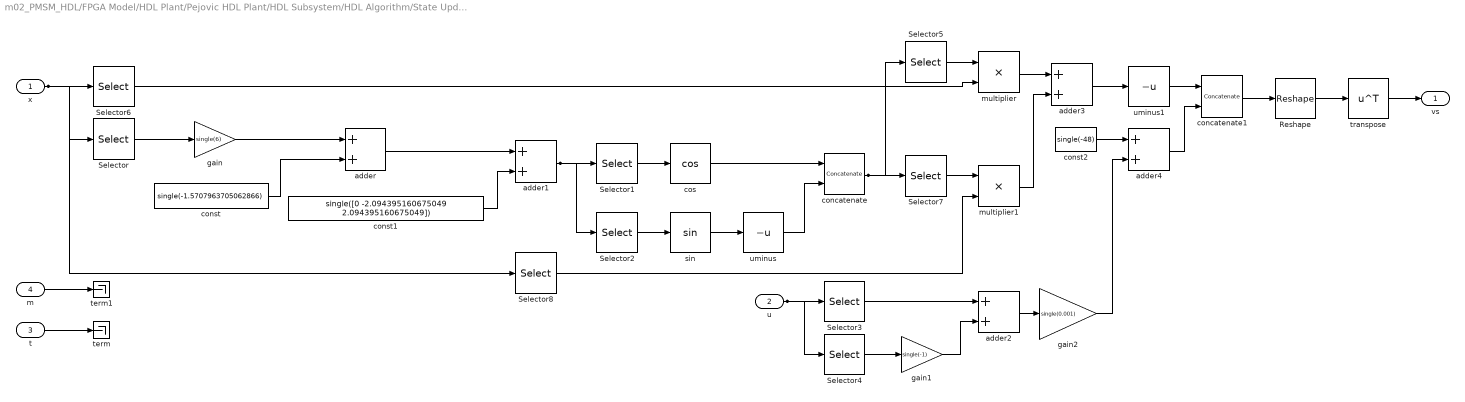
== system m02_PMSM_HDL/FPGA Model/HDL Plant/Pejovic HDL Plant/HDL Subsystem/HDL Algorithm/State Update/Algebraic Clump2/extClump1_F ==
  x : Inport  OutDataTypeStr=single  PortDimensions=[5 1]  SampleTime=2.5e-06
  u : Inport  Port=2  OutDataTypeStr=single  PortDimensions=[2 1]  SampleTime=2.5e-06
  t : Inport  Port=3  OutDataTypeStr=single  SampleTime=2.5e-06
  m : Inport  Port=4  OutDataTypeStr=int32  SampleTime=2.5e-06
  Reshape : Reshape  OutputDimensionality=Column vector (2-D)
  Selector : Selector  SampleTime=2.5e-06  IndexOptions=Index vector (dialog)  Indices=double(3)  OutputSizes=double(0)
  Selector1 : Selector  SampleTime=2.5e-06  IndexOptions=Index vector (dialog)  Indices=double(3)  OutputSizes=double(0)
  Selector2 : Selector  SampleTime=2.5e-06  IndexOptions=Index vector (dialog)  Indices=double(3)  OutputSizes=double(0)
  Selector3 : Selector  SampleTime=2.5e-06  IndexOptions=Index vector (dialog)  Indices=double(1)  OutputSizes=double(0)
  Selector4 : Selector  SampleTime=2.5e-06  IndexOptions=Index vector (dialog)  Indices=double(2)  OutputSizes=double(0)
  Selector5 : Selector  SampleTime=2.5e-06  IndexOptions=Index vector (dialog)  Indices=double(1)  OutputSizes=double(0)
  Selector6 : Selector  SampleTime=2.5e-06  IndexOptions=Index vector (dialog)  Indices=double(4)  OutputSizes=double(0)
  Selector7 : Selector  SampleTime=2.5e-06  IndexOptions=Index vector (dialog)  Indices=double(2)  OutputSizes=double(0)
  Selector8 : Selector  SampleTime=2.5e-06  IndexOptions=Index vector (dialog)  Indices=double(5)  OutputSizes=double(0)
  adder{,1..4} (5 alike) : Sum  OutDataTypeStr=single  AccumDataTypeStr=single  SampleTime=2.5e-06
  concatenate : Concatenate  Mode=Multidimensional array  ConcatenateDimension=2
  concatenate1 : Concatenate  Mode=Multidimensional array
  const : Constant  Value=single(-1.5707963705062866)  VectorParams1D=off  OutDataTypeStr=single  SampleTime=2.5e-06
  const1 : Constant  Value=single([0 -2.094395160675049 2.094395160675049])  VectorParams1D=off  OutDataTypeStr=single  SampleTime=2.5e-06
  const2 : Constant  Value=single(-48)  VectorParams1D=off  OutDataTypeStr=single  SampleTime=2.5e-06
  cos : Trigonometry  Operator=cos  SampleTime=2.5e-06
  gain : Gain  Gain=single(6)  OutDataTypeStr=single  SampleTime=2.5e-06
  gain1 : Gain  Gain=single(-1)  OutDataTypeStr=single  SampleTime=2.5e-06
  gain2 : Gain  Gain=single(0.001)  OutDataTypeStr=single  SampleTime=2.5e-06
  multiplier : Product  Inputs=**  OutDataTypeStr=single  SampleTime=2.5e-06
  multiplier1 : Product  Inputs=**  OutDataTypeStr=single  SampleTime=2.5e-06
  sin : Trigonometry  SampleTime=2.5e-06
  term : Terminator
  term1 : Terminator
  transpose : Math  Operator=transpose
  uminus : UnaryMinus  SampleTime=2.5e-06
  uminus1 : UnaryMinus  SampleTime=2.5e-06
  vs : Outport  OutDataTypeStr=single  PortDimensions=[1 2]  SampleTime=2.5e-06
  wires:
  u/1 -> Selector4/1, Selector3/1
  x/1 -> Selector8/1, Selector6/1, Selector/1
  m/1 -> term1/1
  t/1 -> term/1
  cos/1 -> concatenate/1
  gain/1 -> adder/1
  Selector5/1 -> multiplier/1
  Selector6/1 -> multiplier/2
  Reshape/1 -> transpose/1
  Selector/1 -> gain/1
  const2/1 -> adder4/1
  const1/1 -> adder1/2
  const/1 -> adder/2
  adder/1 -> adder1/1
  adder2/1 -> gain2/1
  adder1/1 -> Selector2/1, Selector1/1
  Selector7/1 -> multiplier1/1
  Selector8/1 -> multiplier1/2
  Selector2/1 -> sin/1
  Selector1/1 -> cos/1
  multiplier1/1 -> adder3/2
  sin/1 -> uminus/1
  transpose/1 -> vs/1
  uminus/1 -> concatenate/2
  concatenate1/1 -> Reshape/1
  concatenate/1 -> Selector7/1, Selector5/1
  Selector4/1 -> gain1/1
  Selector3/1 -> adder2/1
  gain2/1 -> adder4/2
  gain1/1 -> adder2/2
  multiplier/1 -> adder3/1
  adder3/1 -> uminus1/1
  uminus1/1 -> concatenate1/1
  adder4/1 -> concatenate1/2

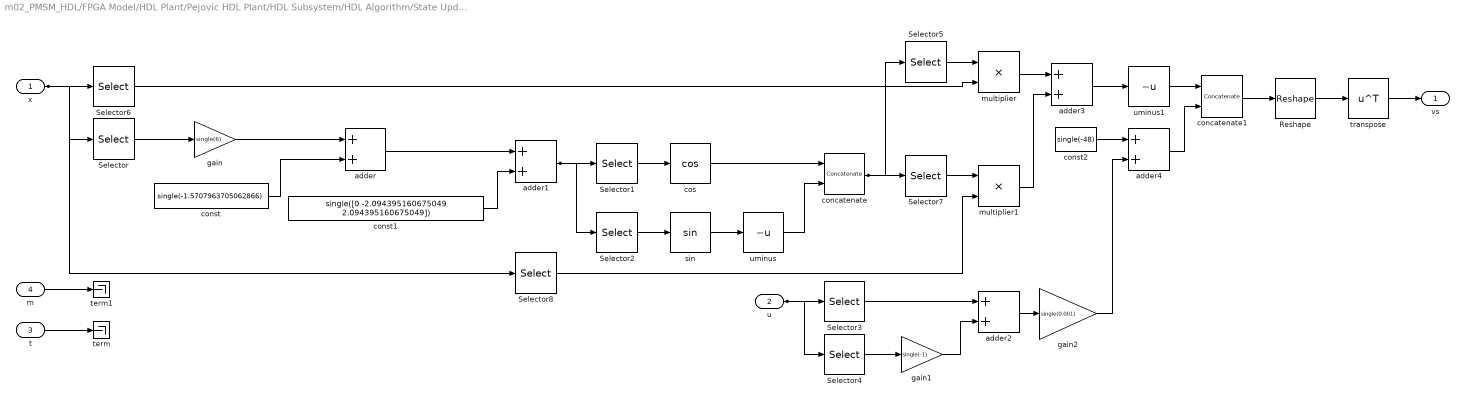
== system m02_PMSM_HDL/FPGA Model/HDL Plant/Pejovic HDL Plant/HDL Subsystem/HDL Algorithm/State Update/Algebraic Clump3/extClump2_F ==
  x : Inport  OutDataTypeStr=single  PortDimensions=[5 1]  SampleTime=2.5e-06
  u : Inport  Port=2  OutDataTypeStr=single  PortDimensions=[2 1]  SampleTime=2.5e-06
  t : Inport  Port=3  OutDataTypeStr=single  SampleTime=2.5e-06
  m : Inport  Port=4  OutDataTypeStr=int32  SampleTime=2.5e-06
  Reshape : Reshape  OutputDimensionality=Column vector (2-D)
  Selector : Selector  SampleTime=2.5e-06  IndexOptions=Index vector (dialog)  Indices=double(3)  OutputSizes=double(0)
  Selector{1..2,4,7} (4 alike) : Selector  SampleTime=2.5e-06  IndexOptions=Index vector (dialog)  Indices=double(2)  OutputSizes=double(0)
  Selector3 : Selector  SampleTime=2.5e-06  IndexOptions=Index vector (dialog)  Indices=double(1)  OutputSizes=double(0)
  Selector5 : Selector  SampleTime=2.5e-06  IndexOptions=Index vector (dialog)  Indices=double(1)  OutputSizes=double(0)
  Selector6 : Selector  SampleTime=2.5e-06  IndexOptions=Index vector (dialog)  Indices=double(4)  OutputSizes=double(0)
  Selector8 : Selector  SampleTime=2.5e-06  IndexOptions=Index vector (dialog)  Indices=double(5)  OutputSizes=double(0)
  adder{,1..4} (5 alike) : Sum  OutDataTypeStr=single  AccumDataTypeStr=single  SampleTime=2.5e-06
  concatenate : Concatenate  Mode=Multidimensional array  ConcatenateDimension=2
  concatenate1 : Concatenate  Mode=Multidimensional array
  const : Constant  Value=single(-1.5707963705062866)  VectorParams1D=off  OutDataTypeStr=single  SampleTime=2.5e-06
  const1 : Constant  Value=single([0 -2.094395160675049 2.094395160675049])  VectorParams1D=off  OutDataTypeStr=single  SampleTime=2.5e-06
  const2 : Constant  Value=single(-48)  VectorParams1D=off  OutDataTypeStr=single  SampleTime=2.5e-06
  cos : Trigonometry  Operator=cos  SampleTime=2.5e-06
  gain : Gain  Gain=single(6)  OutDataTypeStr=single  SampleTime=2.5e-06
  gain1 : Gain  Gain=single(-1)  OutDataTypeStr=single  SampleTime=2.5e-06
  gain2 : Gain  Gain=single(0.001)  OutDataTypeStr=single  SampleTime=2.5e-06
  multiplier : Product  Inputs=**  OutDataTypeStr=single  SampleTime=2.5e-06
  multiplier1 : Product  Inputs=**  OutDataTypeStr=single  SampleTime=2.5e-06
  sin : Trigonometry  SampleTime=2.5e-06
  term : Terminator
  term1 : Terminator
  transpose : Math  Operator=transpose
  uminus : UnaryMinus  SampleTime=2.5e-06
  uminus1 : UnaryMinus  SampleTime=2.5e-06
  vs : Outport  OutDataTypeStr=single  PortDimensions=[1 2]  SampleTime=2.5e-06
  wires:
  x/1 -> Selector8/1, Selector6/1, Selector/1
  Reshape/1 -> transpose/1
  m/1 -> term1/1
  u/1 -> Selector4/1, Selector3/1
  t/1 -> term/1
  gain1/1 -> adder2/2
  gain/1 -> adder/1
  Selector7/1 -> multiplier1/1
  Selector6/1 -> multiplier/2
  Selector1/1 -> cos/1
  Selector/1 -> gain/1
  concatenate1/1 -> Reshape/1
  const1/1 -> adder1/2
  const/1 -> adder/2
  Selector8/1 -> multiplier1/2
  adder/1 -> adder1/1
  adder1/1 -> Selector2/1, Selector1/1
  Selector3/1 -> adder2/1
  Selector2/1 -> sin/1
  const2/1 -> adder4/1
  cos/1 -> concatenate/1
  transpose/1 -> vs/1
  sin/1 -> uminus/1
  uminus1/1 -> concatenate1/1
  uminus/1 -> concatenate/2
  concatenate/1 -> Selector7/1, Selector5/1
  Selector5/1 -> multiplier/1
  Selector4/1 -> gain1/1
  gain2/1 -> adder4/2
  multiplier/1 -> adder3/1
  multiplier1/1 -> adder3/2
  adder2/1 -> gain2/1
  adder4/1 -> concatenate1/2
  adder3/1 -> uminus1/1
